simulink library "csr"  (Simulink 8.1)
settings: Solver=ode1  StartTime=0.0  StopTime=Inf  FixedStep=0.001  RelTol=1e-3
PostLoadFcn:
  | , if any(exist('dsrtsu_mdlpostloadfcn', 'file') == [2, 3, 6]), try dsrtsu_mdlpostloadfcn('Execute', bdroot); catch fprintf('Error in PostLoadFcn (dsrtsu_mdlpostloadfcn) for model "%s":\n %s\n', bdroot, lasterr); end, end,
undefined symbols (not defined in the file or in its folder): FALSE, KJUD_ACCMaxActSpeed_kph, KJUD_ACCMaxDeactSpeed_kph, KJUD_ACCMinActSpeed_kph, KJUD_ACCMinDeactSpeed_kph, TRUE
settings Model: DSRTSU_INTERNAL_RTI_VER=450  DSRTSU_INTERNAL_RTI_TYPE=rti1401  RTICANMMDATA=struct('GeneralSetupData',struct('modelroot','D:\ELN150201_TAIWAN\trunk\AdasDragon\software\sw_development\arch\app\jud','generalsettings',struct('filesettings',struct('destfolder',struct('Name','RTICANMM_FILES','Check',1),'buildfolder',struct('Name','.','Check',1),'AbsDestfolder',struct('Name','D:\ELN150201_TAIWAN\trunk\AdasDragon\software\sw_development\arch\app\jud\RTICANMM_FILES'),'AbsBuildfolder',struct('Name','D:\ELN150201_TAIWAN\trunk\AdasDragon\software\sw_development\arch\app\jud'))),'options',struct('addpaths',1,'rmpaths',1,'addtrcexclusion',logical(1),'cannavigator',struct('checkmonitoring',0),'show_usrtrc',0,'use_usrtrc',0),'advanced',struct('options',[1 1 1 1 1 1 1 1 1 1 1 1 1 1 1 1 1 1 1 1 1 1 1 1 1 1 1 1 1 1 1 1 1 1 1 1 1 1 1 1 1 1 1 1 1 1 1 1 1 1 1 1 1 1 1 1 1 1 1 1 1 1 1 1 1 1 1 1 1 1 1 1 1 1 1 1 1 1 1 1 1 1 1 1 1 1 1 1 1 1 1 1 1 1 1 1 1 1 1 1]),'MPSetup',{{}},'modelname','csr','block','csr'))  DSRTSU_INTERNAL_RTIFPGA=40  Creator=AT015411  LastModifiedBy=AT015555

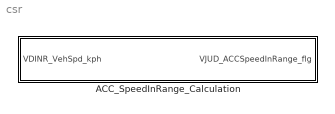
== system csr ==
  ACC_SpeedInRange_Calculation : Subsystem

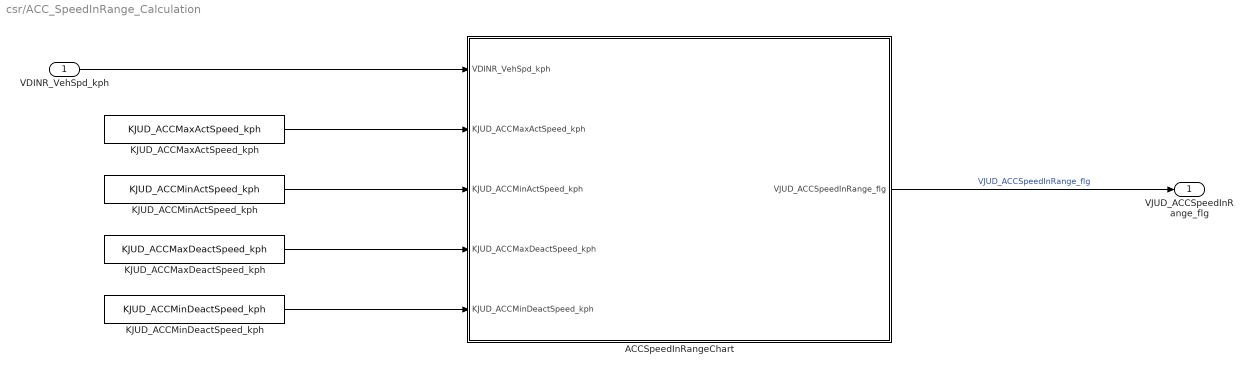
== system csr/ACC_SpeedInRange_Calculation ==
  VDINR_VehSpd_kph : Inport
  ACCSpeedInRangeChart : Stateflow chart  TreatAsAtomicUnit=on
  KJUD_ACCMaxActSpeed_kph : Constant  Value=KJUD_ACCMaxActSpeed_kph
  KJUD_ACCMaxDeactSpeed_kph : Constant  Value=KJUD_ACCMaxDeactSpeed_kph
  KJUD_ACCMinActSpeed_kph : Constant  Value=KJUD_ACCMinActSpeed_kph
  KJUD_ACCMinDeactSpeed_kph : Constant  Value=KJUD_ACCMinDeactSpeed_kph
  VJUD_ACCSpeedInRange_flg : Outport
  wires:
  KJUD_ACCMaxActSpeed_kph/1 -> ACCSpeedInRangeChart/2(KJUD_ACCMaxActSpeed_kph)
  KJUD_ACCMinActSpeed_kph/1 -> ACCSpeedInRangeChart/3(KJUD_ACCMinActSpeed_kph)
  ACCSpeedInRangeChart/1(VJUD_ACCSpeedInRange_flg) -> VJUD_ACCSpeedInRange_flg/1  "VJUD_ACCSpeedInRange_flg"
  VDINR_VehSpd_kph/1 -> ACCSpeedInRangeChart/1(VDINR_VehSpd_kph)
  KJUD_ACCMaxDeactSpeed_kph/1 -> ACCSpeedInRangeChart/4(KJUD_ACCMaxDeactSpeed_kph)
  KJUD_ACCMinDeactSpeed_kph/1 -> ACCSpeedInRangeChart/5(KJUD_ACCMinDeactSpeed_kph)

== stateflow chart ACC_SpeedInRange_Calculation/ACCSpeedInRangeChart ==
  state SPEED_OUT_OF_RANGE
    en:
    VJUD_ACCSpeedInRange_flg=FALSE;
  state SPEED_IN_RANGE
    en:
    VJUD_ACCSpeedInRange_flg=TRUE;
  (default) -> SPEED_OUT_OF_RANGE
  SPEED_OUT_OF_RANGE -> SPEED_IN_RANGE : [(VDINR_VehSpd_kph>=KJUD_ACCMinActSpeed_kph)...
      | &&(VDINR_VehSpd_kph<=KJUD_ACCMaxActSpeed_kph)]
  SPEED_IN_RANGE -> SPEED_OUT_OF_RANGE : [(VDINR_VehSpd_kph<=KJUD_ACCMinDeactSpeed_kph)...
      | ||(VDINR_VehSpd_kph>=KJUD_ACCMaxDeactSpeed_kph)]
  data: VDINR_VehSpd_kph input single; VJUD_ACCSpeedInRange_flg output boolean; FALSE parameter boolean; TRUE parameter boolean; KJUD_ACCMaxActSpeed_kph input single; KJUD_ACCMinActSpeed_kph input single; KJUD_ACCMaxDeactSpeed_kph input single; KJUD_ACCMinDeactSpeed_kph input single
